simulink model "IEEE34_PQload"  (R2021b)
settings: Solver=ode4  StartTime=0.0  StopTime=5  FixedStep=50e-6  RelTol=1e-3
PreLoadFcn:
  | pGain = 0.05; % Gain of random perturbation (pu)
  | pGainAP = 0.01; % Gain of sinusoidal active power variation (pu)
  | pGainRP = 0.01; % Gain of sinusoidal reactive power variation (pu)
  | pFreqAP = 0.03; % Frequency of sinusoidal active power variation (Hz)
  | pFreqRP = 0.03; % Frequency of sinusoidal reactive power variation (Hz)
  | 
  | init_IEEE34nodetestfeeder;
InitFcn:
  | pGain = 0.05; % Gain of random perturbation (pu)
  | pGainAP = 0.01; % Gain of sinusoidal active power variation (pu)
  | pGainRP = 0.01; % Gain of sinusoidal reactive power variation (pu)
  | pFreqAP = 0.03; % Frequency of sinusoidal active power variation (Hz)
  | pFreqRP = 0.03; % Frequency of sinusoidal reactive power variation (Hz)
  | 
  | init_IEEE34nodetestfeeder;
values from neighbouring files (symbols this model uses):
  fNom = f    (= 60)    [init_IEEE34nodetestfeeder.m]
  loadcoeff = 1.0    (= 1)    [init_IEEE34nodetestfeeder.m]
  Pbase = 500e3    (= 500000)    [init_IEEE34nodetestfeeder.m]
  Ts = 50e-6    (= 5e-05)    [init_IEEE34nodetestfeeder.m]
  vNomMV = VsubL    (= 24900)    [init_IEEE34nodetestfeeder.m]
  VsubL = 24.9e3    (= 24900)    [init_IEEE34nodetestfeeder.m]
undefined symbols (not defined in the file or in its folder): find_system
libraries: spsSeriesRLCBranchLib x330, spsGroundLib x242, LoadLib x88, spsThreePhaseVIMeasurementLib x37, spsMutualInductanceLib x24, spsVoltageMeasurementLib x18, spsCurrentMeasurementLib x12, spsOnDelayLib x12, spsRMSLib x8, spsLinearTransformerLib x6, spsControlledCurrentSourceLib x6, spsControlledVoltageSourceLib x6
(part 1 of 8)
settings Model: ARTEMISmethode_block_infos=$$__separator__$$  Creator=hosseinh  LastModifiedBy=gl8300
settings SolverCC: AlgebraicLoopSolver=TrustRegion  AutoInsertRateTranBlk=on  InsertRTBMode=Never (minimum delay)
settings DataIOCC: LimitDataPoints=on  SaveFormat=Array  SignalLoggingSaveFormat=ModelDataLogs  SaveOutput=off  SignalLogging=off  DSMLogging=off  SaveTime=off  ReturnWorkspaceOutputs=off
settings OptimizationCC: BlockReduction=off  ExpressionDepthLimit=2147483647  LifeSpan=inf
settings DebuggingCC: UnderspecifiedInitializationDetection=Classic  MergeDetectMultiDrivingBlocksExec=none  SolverPrmCheckMsg=warning  FcnCallInpInsideContextMsg=warning  AllowSymbolicDim=off  StateNameClashWarn=warning  SFUnexpectedBacktrackingDiag=warning  SFNoUnconditionalDefaultTransitionDiag=warning  SFExecutionAtInitializationDiag=none  SFMachineParentedDataDiag=warning  ArithmeticOperatorsInVariantConditions=warning
settings HardwareCC: ProdBitPerPointer=32  ProdBitPerSizeT=32  ProdBitPerPtrDiffT=32  ProdLargestAtomicFloat=None  ProdIntDivRoundTo=Undefined  ProdEndianess=Unspecified  ProdWordSize=32  ProdHWDeviceType=32-bit Generic
settings ModelReferenceCC: PropagateSignalLabelsOutOfModel=off
settings SFSimCC: SimUseLocalCustomCode=off  CustomCodeUndefinedFunction=UseInterfaceOnly
settings RTWCC: RTWUseLocalCustomCode=off
settings CodeAppCC: StateflowObjectComments=on
settings GRTTargetCC: TargetLangStandard=C89/C90 (ANSI)  CombineOutputUpdateFcns=off  GRTInterface=on
settings ConfigComp: CovMetricSettings=dw  CovSaveCumulativeToWorkspaceVar=on  CovSaveSingleToWorkspaceVar=on  CovExternalEMLEnable=off
settings SimscapeCC: SimscapeNormalizeSystem=off

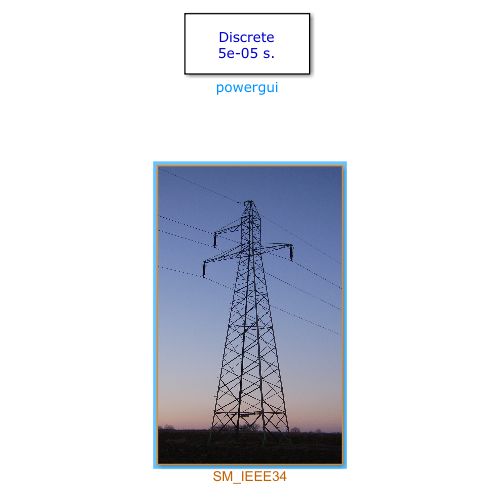
[thumbnail: Simulink's stored preview of the top-level diagram]
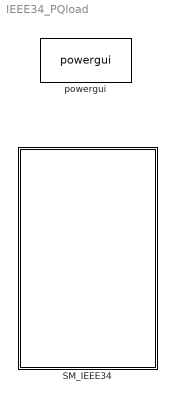
== system IEEE34_PQload ==
  SM_IEEE34 : Subsystem
      mask Display: image(imread('MVT.jpg'))
  powergui : spspowerguiLib/powergui  Priority=1  SimulationMode=Discrete  SampleTime=Ts  frequency=60  Iterations=50  frequencyindice=0  Pbase=100e6  ErrMax=1e-4  UnitsV=kV  UnitsW=MW  buscounter=0  FunctionMessages=off  echomessages=on  EnableUseOfTLC=off  CurrentSourceSwitches=off  DisableSnubberDevices=off  DisableRonSwitches=off  DisableVfSwitches=off  DisplayEquations=off  AutomaticDiscreteSolvers=off  SolverType=Backward Euler  Interpol=off  ExternalGateDelay=off  methode=off  Ts=0  x0status=blocks  SPID=off  SwTol=0  HookPort=off  NonlinearTolerance=1e-4  nMaxIteration=100  ContinueOnMaxIteration=off  RestoreLinks=warning  ResistiveCurrentMeasurement=off  Frange=[0:2:500]  Ylog=off  Xlog=on  ShowGrid=off  save=off  variable=ZData  structure=0  ZoomFFT=off  StartTime=0.0  cycles=1  DisplayStyle=1  fundamental=60  FreqAxis=off  MaxFrequency=1000  frequencyindicesteady=1  RmsSteady=1  display=off

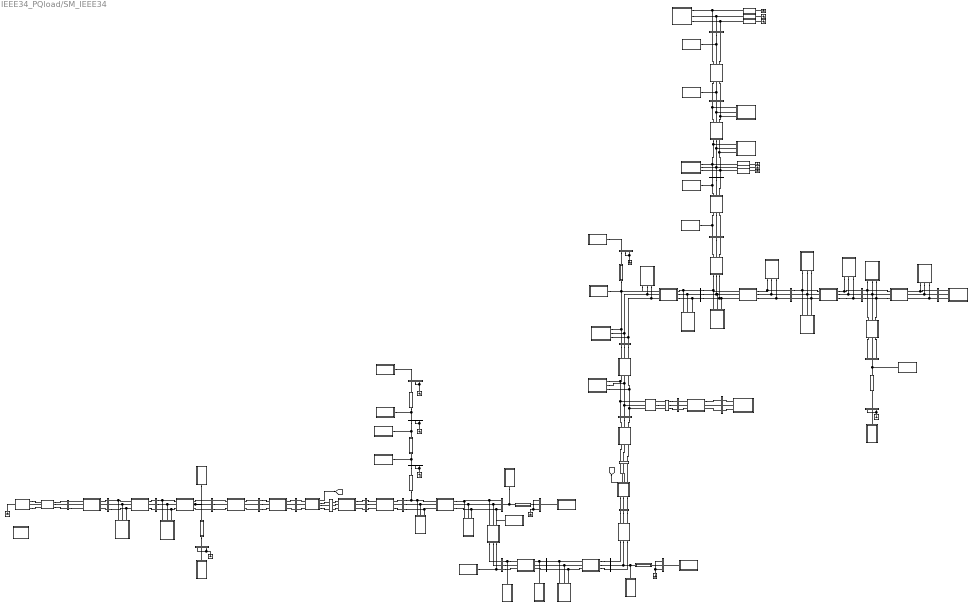
== system IEEE34_PQload/SM_IEEE34 ==
  note: Y-Z
  note: Y-PQ
  note: Y-I
  note: Y-PQ
  note: D-I
  note: Y-PQ
  note: Y-PQ
  note: Y-PQ
  note: Y-PQ
  note: D-PQ
  note: D-I
  note: Y-PQ
  note: Y-PQ
  note: Y-PQ
  note: D-I
  note: D-Z
  note: D-I
  note: Y-PQ
  note: D-PQ
  note: Y-I
  note: Y-I
  note: Y-PQ
  note: Y-Z
  800 : spsThreePhaseVIMeasurementLib/Three-Phase V-I Measurement  VoltageMeasurement=phase-to-ground  SetLabelV=on  LabelV=Vabc_800  Vpu=off  VpuLL=off  CurrentMeasurement=yes  SetLabelI=on  LabelI=Iabc_800  Ipu=off  Pbase=Pbase  Vbase=Vbase  OutputType=Complex  PhasorSimulation=off  PSBequivalent=0
  802 : spsThreePhaseVIMeasurementLib/Three-Phase V-I Measurement  VoltageMeasurement=phase-to-ground  SetLabelV=on  LabelV=Vabc_802  Vpu=off  VpuLL=off  CurrentMeasurement=yes  SetLabelI=on  LabelI=Iabc_802  Ipu=off  Pbase=Pbase  Vbase=Vbase  OutputType=Complex  PhasorSimulation=off  PSBequivalent=0
  806 : spsThreePhaseVIMeasurementLib/Three-Phase V-I Measurement  VoltageMeasurement=phase-to-ground  SetLabelV=on  LabelV=Vabc_806  Vpu=off  VpuLL=off  CurrentMeasurement=yes  SetLabelI=on  LabelI=Iabc_806  Ipu=off  Pbase=Pbase  Vbase=Vbase  OutputType=Complex  PhasorSimulation=off  PSBequivalent=0
  808 : spsThreePhaseVIMeasurementLib/Three-Phase V-I Measurement  VoltageMeasurement=phase-to-ground  SetLabelV=on  LabelV=Vabc_808  Vpu=off  VpuLL=off  CurrentMeasurement=yes  SetLabelI=on  LabelI=Iabc_808  Ipu=off  Pbase=Pbase  Vbase=Vbase  OutputType=Complex  PhasorSimulation=off  PSBequivalent=0
  810 : spsThreePhaseVIMeasurementLib/Three-Phase V-I Measurement  VoltageMeasurement=phase-to-ground  SetLabelV=on  LabelV=Vabc_810  Vpu=off  VpuLL=off  CurrentMeasurement=yes  SetLabelI=on  LabelI=Iabc_810  Ipu=off  Pbase=Pbase  Vbase=Vbase  OutputType=Complex  PhasorSimulation=off  PSBequivalent=0
  812 : spsThreePhaseVIMeasurementLib/Three-Phase V-I Measurement  VoltageMeasurement=phase-to-ground  SetLabelV=on  LabelV=Vabc_812  Vpu=off  VpuLL=off  CurrentMeasurement=yes  SetLabelI=on  LabelI=Iabc_812  Ipu=off  Pbase=Pbase  Vbase=Vbase  OutputType=Complex  PhasorSimulation=off  PSBequivalent=0
  814 : spsThreePhaseVIMeasurementLib/Three-Phase V-I Measurement  VoltageMeasurement=phase-to-ground  SetLabelV=on  LabelV=Vabc_814  Vpu=off  VpuLL=off  CurrentMeasurement=yes  SetLabelI=on  LabelI=Iabc_814  Ipu=off  Pbase=Pbase  Vbase=Vbase  OutputType=Complex  PhasorSimulation=off  PSBequivalent=0
  816 : spsThreePhaseVIMeasurementLib/Three-Phase V-I Measurement  VoltageMeasurement=phase-to-ground  SetLabelV=on  LabelV=Vabc_816  Vpu=off  VpuLL=off  CurrentMeasurement=yes  SetLabelI=on  LabelI=Iabc_816  Ipu=off  Pbase=Pbase  Vbase=Vbase  OutputType=Complex  PhasorSimulation=off  PSBequivalent=0
  818 : spsThreePhaseVIMeasurementLib/Three-Phase V-I Measurement  VoltageMeasurement=phase-to-ground  SetLabelV=on  LabelV=Vabc_818  Vpu=off  VpuLL=off  CurrentMeasurement=yes  SetLabelI=on  LabelI=Iabc_818  Ipu=off  Pbase=Pbase  Vbase=Vbase  OutputType=Complex  PhasorSimulation=off  PSBequivalent=0
  820 : spsThreePhaseVIMeasurementLib/Three-Phase V-I Measurement  VoltageMeasurement=phase-to-ground  SetLabelV=on  LabelV=Vabc_820  Vpu=off  VpuLL=off  CurrentMeasurement=yes  SetLabelI=on  LabelI=Iabc_820  Ipu=off  Pbase=Pbase  Vbase=Vbase  OutputType=Complex  PhasorSimulation=off  PSBequivalent=0
  822 : spsThreePhaseVIMeasurementLib/Three-Phase V-I Measurement  VoltageMeasurement=phase-to-ground  SetLabelV=on  LabelV=Vabc_822  Vpu=off  VpuLL=off  CurrentMeasurement=yes  SetLabelI=on  LabelI=Iabc_822  Ipu=off  Pbase=Pbase  Vbase=Vbase  OutputType=Complex  PhasorSimulation=off  PSBequivalent=0
  824 : spsThreePhaseVIMeasurementLib/Three-Phase V-I Measurement  VoltageMeasurement=phase-to-ground  SetLabelV=on  LabelV=Vabc_824  Vpu=off  VpuLL=off  CurrentMeasurement=yes  SetLabelI=on  LabelI=Iabc_824  Ipu=off  Pbase=Pbase  Vbase=Vbase  OutputType=Complex  PhasorSimulation=off  PSBequivalent=0
  826 : spsThreePhaseVIMeasurementLib/Three-Phase V-I Measurement  VoltageMeasurement=phase-to-ground  SetLabelV=on  LabelV=Vabc_826  Vpu=off  VpuLL=off  CurrentMeasurement=yes  SetLabelI=on  LabelI=Iabc_826  Ipu=off  Pbase=Pbase  Vbase=Vbase  OutputType=Complex  PhasorSimulation=off  PSBequivalent=0
  828 : spsThreePhaseVIMeasurementLib/Three-Phase V-I Measurement  VoltageMeasurement=phase-to-ground  SetLabelV=on  LabelV=Vabc_828  Vpu=off  VpuLL=off  CurrentMeasurement=yes  SetLabelI=on  LabelI=Iabc_828  Ipu=off  Pbase=Pbase  Vbase=Vbase  OutputType=Complex  PhasorSimulation=off  PSBequivalent=0
  830 : spsThreePhaseVIMeasurementLib/Three-Phase V-I Measurement  VoltageMeasurement=phase-to-ground  SetLabelV=on  LabelV=Vabc_830  Vpu=off  VpuLL=off  CurrentMeasurement=yes  SetLabelI=on  LabelI=Iabc_830  Ipu=off  Pbase=Pbase  Vbase=Vbase  OutputType=Complex  PhasorSimulation=off  PSBequivalent=0
  832 : spsThreePhaseVIMeasurementLib/Three-Phase V-I Measurement  VoltageMeasurement=phase-to-ground  SetLabelV=on  LabelV=Vabc_832  Vpu=off  VpuLL=off  CurrentMeasurement=yes  SetLabelI=on  LabelI=Iabc_832  Ipu=off  Pbase=Pbase  Vbase=Vbase  OutputType=Complex  PhasorSimulation=off  PSBequivalent=0
  834 : spsThreePhaseVIMeasurementLib/Three-Phase V-I Measurement  VoltageMeasurement=phase-to-ground  SetLabelV=on  LabelV=Vabc_834  Vpu=off  VpuLL=off  CurrentMeasurement=yes  SetLabelI=on  LabelI=Iabc_834  Ipu=off  Pbase=Pbase  Vbase=Vbase  OutputType=Complex  PhasorSimulation=off  PSBequivalent=0
  836 : spsThreePhaseVIMeasurementLib/Three-Phase V-I Measurement  VoltageMeasurement=phase-to-ground  SetLabelV=on  LabelV=Vabc_836  Vpu=off  VpuLL=off  CurrentMeasurement=yes  SetLabelI=on  LabelI=Iabc_836  Ipu=off  Pbase=Pbase  Vbase=Vbase  OutputType=Complex  PhasorSimulation=off  PSBequivalent=0
  838 : spsThreePhaseVIMeasurementLib/Three-Phase V-I Measurement  VoltageMeasurement=phase-to-ground  SetLabelV=on  LabelV=Vabc_838  Vpu=off  VpuLL=off  CurrentMeasurement=yes  SetLabelI=on  LabelI=Iabc_838  Ipu=off  Pbase=Pbase  Vbase=Vbase  OutputType=Complex  PhasorSimulation=off  PSBequivalent=0
  840 : spsThreePhaseVIMeasurementLib/Three-Phase V-I Measurement  VoltageMeasurement=phase-to-ground  SetLabelV=on  LabelV=Vabc_840  Vpu=off  VpuLL=off  CurrentMeasurement=yes  SetLabelI=on  LabelI=Iabc_840  Ipu=off  Pbase=Pbase  Vbase=Vbase  OutputType=Complex  PhasorSimulation=off  PSBequivalent=0
  842 : spsThreePhaseVIMeasurementLib/Three-Phase V-I Measurement  VoltageMeasurement=phase-to-ground  SetLabelV=on  LabelV=Vabc_842  Vpu=off  VpuLL=off  CurrentMeasurement=yes  SetLabelI=on  LabelI=Iabc_842  Ipu=off  Pbase=Pbase  Vbase=Vbase  OutputType=Complex  PhasorSimulation=off  PSBequivalent=0
  844 : spsThreePhaseVIMeasurementLib/Three-Phase V-I Measurement  VoltageMeasurement=phase-to-ground  SetLabelV=on  LabelV=Vabc_844  Vpu=off  VpuLL=off  CurrentMeasurement=yes  SetLabelI=on  LabelI=Iabc_844  Ipu=off  Pbase=Pbase  Vbase=Vbase  OutputType=Complex  PhasorSimulation=off  PSBequivalent=0
  846 : spsThreePhaseVIMeasurementLib/Three-Phase V-I Measurement  VoltageMeasurement=phase-to-ground  SetLabelV=on  LabelV=Vabc_846  Vpu=off  VpuLL=off  CurrentMeasurement=yes  SetLabelI=on  LabelI=Iabc_846  Ipu=off  Pbase=Pbase  Vbase=Vbase  OutputType=Complex  PhasorSimulation=off  PSBequivalent=0
  848 : spsThreePhaseVIMeasurementLib/Three-Phase V-I Measurement  VoltageMeasurement=phase-to-ground  SetLabelV=on  LabelV=Vabc_848  Vpu=off  VpuLL=off  CurrentMeasurement=yes  SetLabelI=on  LabelI=Iabc_848  Ipu=off  Pbase=Pbase  Vbase=Vbase  OutputType=Complex  PhasorSimulation=off  PSBequivalent=0
  850 : spsThreePhaseVIMeasurementLib/Three-Phase V-I Measurement  VoltageMeasurement=phase-to-ground  SetLabelV=on  LabelV=Vabc_850  Vpu=off  VpuLL=off  CurrentMeasurement=yes  SetLabelI=on  LabelI=Iabc_850  Ipu=off  Pbase=Pbase  Vbase=Vbase  OutputType=Complex  PhasorSimulation=off  PSBequivalent=0
  "852 " : spsThreePhaseVIMeasurementLib/Three-Phase V-I Measurement  VoltageMeasurement=phase-to-ground  SetLabelV=on  LabelV=Vabc_852  Vpu=off  VpuLL=off  CurrentMeasurement=yes  SetLabelI=on  LabelI=Iabc_852  Ipu=off  Pbase=100e6  Vbase=24900  OutputType=Complex  PhasorSimulation=off  PSBequivalent=0
  854 : spsThreePhaseVIMeasurementLib/Three-Phase V-I Measurement  VoltageMeasurement=phase-to-ground  SetLabelV=on  LabelV=Vabc_854  Vpu=off  VpuLL=off  CurrentMeasurement=yes  SetLabelI=on  LabelI=Iabc_854  Ipu=off  Pbase=Pbase  Vbase=Vbase  OutputType=Complex  PhasorSimulation=off  PSBequivalent=0
  856 : spsThreePhaseVIMeasurementLib/Three-Phase V-I Measurement  VoltageMeasurement=phase-to-ground  SetLabelV=on  LabelV=Vabc_856  Vpu=off  VpuLL=off  CurrentMeasurement=yes  SetLabelI=on  LabelI=Iabc_856  Ipu=off  Pbase=Pbase  Vbase=Vbase  OutputType=Complex  PhasorSimulation=off  PSBequivalent=0
  858 : spsThreePhaseVIMeasurementLib/Three-Phase V-I Measurement  VoltageMeasurement=phase-to-ground  SetLabelV=on  LabelV=Vabc_858  Vpu=off  VpuLL=off  CurrentMeasurement=yes  SetLabelI=on  LabelI=Iabc_858  Ipu=off  Pbase=Pbase  Vbase=Vbase  OutputType=Complex  PhasorSimulation=off  PSBequivalent=0
  860 : spsThreePhaseVIMeasurementLib/Three-Phase V-I Measurement  VoltageMeasurement=phase-to-ground  SetLabelV=on  LabelV=Vabc_860  Vpu=off  VpuLL=off  CurrentMeasurement=yes  SetLabelI=on  LabelI=Iabc_860  Ipu=off  Pbase=Pbase  Vbase=Vbase  OutputType=Complex  PhasorSimulation=off  PSBequivalent=0
  862 : spsThreePhaseVIMeasurementLib/Three-Phase V-I Measurement  VoltageMeasurement=phase-to-ground  SetLabelV=on  LabelV=Vabc_862  Vpu=off  VpuLL=off  CurrentMeasurement=yes  SetLabelI=on  LabelI=Iabc_862  Ipu=off  Pbase=Pbase  Vbase=Vbase  OutputType=Complex  PhasorSimulation=off  PSBequivalent=0
  864 : spsThreePhaseVIMeasurementLib/Three-Phase V-I Measurement  VoltageMeasurement=phase-to-ground  SetLabelV=on  LabelV=Vabc_864  Vpu=off  VpuLL=off  CurrentMeasurement=yes  SetLabelI=on  LabelI=Iabc_864  Ipu=off  Pbase=Pbase  Vbase=Vbase  OutputType=Complex  PhasorSimulation=off  PSBequivalent=0
  888 : spsThreePhaseVIMeasurementLib/Three-Phase V-I Measurement  VoltageMeasurement=phase-to-ground  SetLabelV=on  LabelV=Vabc_888  Vpu=off  VpuLL=off  CurrentMeasurement=yes  SetLabelI=on  LabelI=Iabc_888  Ipu=off  Pbase=Pbase  Vbase=VxfmL  OutputType=Complex  PhasorSimulation=off  PSBequivalent=0
  890 : spsThreePhaseVIMeasurementLib/Three-Phase V-I Measurement  VoltageMeasurement=phase-to-ground  SetLabelV=on  LabelV=Vabc_890  Vpu=off  VpuLL=off  CurrentMeasurement=yes  SetLabelI=on  LabelI=Iabc_890  Ipu=off  Pbase=Pbase  Vbase=VxfmL  OutputType=Complex  PhasorSimulation=off  PSBequivalent=0
  Config1 : Subsystem  mask(Config302 (IEEE 34 Node Test Feeder)){fNom=fNom, length=1.6 * 48150 / 5280}
      mask prompts: fNom "Nominal frequency (Hz)"; length "Length (km)"
      mask Display:
      | patch([20 20 80 80], [30 70 70 30])
      | patch([0 0 20 20], [47 53 53 47])
      | patch([80 80 100 100], [47 53 53 47])
  Config10 : Subsystem  mask(Config300 (IEEE 34 Node Test Feeder)){fNom=fNom, length=1.6 * 29730 / 5280}
      mask prompts: fNom "Nominal frequency (Hz)"; length "Length (km)"
      mask Display:
      | patch([20 20 80 80], [0 20 20 0])
      | patch([0 0 20 20], [7 13 13 7])
      | patch([80 80 100 100], [7 13 13 7])
      | 
      | patch([20 20 80 80], [40 60 60 40])
      | patch([0 0 20 20], [47 53 53 47])
      | patch([80 80 100 100], [47 53 53 47])
      | 
      | patch([20 20 80 80], [80 100 100 80])
      | patch([0 0 20 20], [87 93 93 87])
      | patch([80 80 100 100], [87 93 93 87])
  Config11 : Subsystem  mask(Config301 (IEEE 34 Node Test Feeder)){fNom=fNom, length=1.6 * 310 / 5280}
      mask prompts: fNom "Nominal frequency (Hz)"; length "Length (km)"
      mask Display:
      | patch([20 20 80 80], [0 20 20 0])
      | patch([0 0 20 20], [7 13 13 7])
      | patch([80 80 100 100], [7 13 13 7])
      | 
      | patch([20 20 80 80], [40 60 60 40])
      | patch([0 0 20 20], [47 53 53 47])
      | patch([80 80 100 100], [47 53 53 47])
      | 
      | patch([20 20 80 80], [80 100 100 80])
      | patch([0 0 20 20], [87 93 93 87])
      | patch([80 80 100 100], [87 93 93 87])
  Config12 : Subsystem  mask(Config301 (IEEE 34 Node Test Feeder)){fNom=fNom, length=1.6 * 10210 / 5280}
      mask prompts: fNom "Nominal frequency (Hz)"; length "Length (km)"
      mask Display:
      | patch([20 20 80 80], [0 20 20 0])
      | patch([0 0 20 20], [7 13 13 7])
      | patch([80 80 100 100], [7 13 13 7])
      | 
      | patch([20 20 80 80], [40 60 60 40])
      | patch([0 0 20 20], [47 53 53 47])
      | patch([80 80 100 100], [47 53 53 47])
      | 
      | patch([20 20 80 80], [80 100 100 80])
      | patch([0 0 20 20], [87 93 93 87])
      | patch([80 80 100 100], [87 93 93 87])
  Config13 : Subsystem  mask(Config300 (IEEE 34 Node Test Feeder)){fNom=fNom, length=1.6 * 10560 / 5280}
      mask prompts: fNom "Nominal frequency (Hz)"; length "Length (km)"
      mask Display:
      | patch([20 20 80 80], [0 20 20 0])
      | patch([0 0 20 20], [7 13 13 7])
      | patch([80 80 100 100], [7 13 13 7])
      | 
      | patch([20 20 80 80], [40 60 60 40])
      | patch([0 0 20 20], [47 53 53 47])
      | patch([80 80 100 100], [47 53 53 47])
      | 
      | patch([20 20 80 80], [80 100 100 80])
      | patch([0 0 20 20], [87 93 93 87])
      | patch([80 80 100 100], [87 93 93 87])
  Config14 : Subsystem  mask(Config301 (IEEE 34 Node Test Feeder)){fNom=fNom, length=1.6 * 20440 / 5280}
      mask prompts: fNom "Nominal frequency (Hz)"; length "Length (km)"
      mask Display:
      | patch([20 20 80 80], [0 20 20 0])
      | patch([0 0 20 20], [7 13 13 7])
      | patch([80 80 100 100], [7 13 13 7])
      | 
      | patch([20 20 80 80], [40 60 60 40])
      | patch([0 0 20 20], [47 53 53 47])
      | patch([80 80 100 100], [47 53 53 47])
      | 
      | patch([20 20 80 80], [80 100 100 80])
      | patch([0 0 20 20], [87 93 93 87])
      | patch([80 80 100 100], [87 93 93 87])
  Config15 : Subsystem  mask(Config301 (IEEE 34 Node Test Feeder)){fNom=fNom, length=1.6 * 520 / 5280}
      mask prompts: fNom "Nominal frequency (Hz)"; length "Length (km)"
      mask Display:
      | patch([20 20 80 80], [0 20 20 0])
      | patch([0 0 20 20], [7 13 13 7])
      | patch([80 80 100 100], [7 13 13 7])
      | 
      | patch([20 20 80 80], [40 60 60 40])
      | patch([0 0 20 20], [47 53 53 47])
      | patch([80 80 100 100], [47 53 53 47])
      | 
      | patch([20 20 80 80], [80 100 100 80])
      | patch([0 0 20 20], [87 93 93 87])
      | patch([80 80 100 100], [87 93 93 87])
  Config16 : Subsystem  mask(Config301 (IEEE 34 Node Test Feeder)){fNom=fNom, length=1.6 * 36830 / 5280}
      mask prompts: fNom "Nominal frequency (Hz)"; length "Length (km)"
      mask Display:
      | patch([20 20 80 80], [0 20 20 0])
      | patch([0 0 20 20], [7 13 13 7])
      | patch([80 80 100 100], [7 13 13 7])
      | 
      | patch([20 20 80 80], [40 60 60 40])
      | patch([0 0 20 20], [47 53 53 47])
      | patch([80 80 100 100], [47 53 53 47])
      | 
      | patch([20 20 80 80], [80 100 100 80])
      | patch([0 0 20 20], [87 93 93 87])
      | patch([80 80 100 100], [87 93 93 87])
  Config17 : Subsystem  mask(Config301 (IEEE 34 Node Test Feeder)){fNom=fNom, length=1.6 * 4900 / 5280}
      mask prompts: fNom "Nominal frequency (Hz)"; length "Length (km)"
      mask Display:
      | patch([20 20 80 80], [0 20 20 0])
      | patch([0 0 20 20], [7 13 13 7])
      | patch([80 80 100 100], [7 13 13 7])
      | 
      | patch([20 20 80 80], [40 60 60 40])
      | patch([0 0 20 20], [47 53 53 47])
      | patch([80 80 100 100], [47 53 53 47])
      | 
      | patch([20 20 80 80], [80 100 100 80])
      | patch([0 0 20 20], [87 93 93 87])
      | patch([80 80 100 100], [87 93 93 87])
  Config18 : Subsystem  mask(Config301 (IEEE 34 Node Test Feeder)){fNom=fNom, length=1.6 * 280 / 5280}
      mask prompts: fNom "Nominal frequency (Hz)"; length "Length (km)"
      mask Display:
      | patch([20 20 80 80], [0 20 20 0])
      | patch([0 0 20 20], [7 13 13 7])
      | patch([80 80 100 100], [7 13 13 7])
      | 
      | patch([20 20 80 80], [40 60 60 40])
      | patch([0 0 20 20], [47 53 53 47])
      | patch([80 80 100 100], [47 53 53 47])
      | 
      | patch([20 20 80 80], [80 100 100 80])
      | patch([0 0 20 20], [87 93 93 87])
      | patch([80 80 100 100], [87 93 93 87])
  Config19 : Subsystem  mask(Config301 (IEEE 34 Node Test Feeder)){fNom=fNom, length=1.6 * 1350 / 5280}
      mask prompts: fNom "Nominal frequency (Hz)"; length "Length (km)"
      mask Display:
      | patch([20 20 80 80], [0 20 20 0])
      | patch([0 0 20 20], [7 13 13 7])
      | patch([80 80 100 100], [7 13 13 7])
      | 
      | patch([20 20 80 80], [40 60 60 40])
      | patch([0 0 20 20], [47 53 53 47])
      | patch([80 80 100 100], [47 53 53 47])
      | 
      | patch([20 20 80 80], [80 100 100 80])
      | patch([0 0 20 20], [87 93 93 87])
      | patch([80 80 100 100], [87 93 93 87])
  Config2 : Subsystem  mask(Config302 (IEEE 34 Node Test Feeder)){fNom=fNom, length=1.6 * 13740 / 5280}
      mask prompts: fNom "Nominal frequency (Hz)"; length "Length (km)"
      mask Display:
      | patch([20 20 80 80], [30 70 70 30])
      | patch([0 0 20 20], [47 53 53 47])
      | patch([80 80 100 100], [47 53 53 47])
  Config20 : Subsystem  mask(Config301 (IEEE 34 Node Test Feeder)){fNom=fNom, length=1.6 * 3640 / 5280}
      mask prompts: fNom "Nominal frequency (Hz)"; length "Length (km)"
      mask Display:
      | patch([20 20 80 80], [0 20 20 0])
      | patch([0 0 20 20], [7 13 13 7])
      | patch([80 80 100 100], [7 13 13 7])
      | 
      | patch([20 20 80 80], [40 60 60 40])
      | patch([0 0 20 20], [47 53 53 47])
      | patch([80 80 100 100], [47 53 53 47])
      | 
      | patch([20 20 80 80], [80 100 100 80])
      | patch([0 0 20 20], [87 93 93 87])
      | patch([80 80 100 100], [87 93 93 87])
  Config21 : Subsystem  mask(Config301 (IEEE 34 Node Test Feeder)){fNom=fNom, length=1.6 * 2020 / 5280}
      mask prompts: fNom "Nominal frequency (Hz)"; length "Length (km)"
      mask Display:
      | patch([20 20 80 80], [0 20 20 0])
      | patch([0 0 20 20], [7 13 13 7])
      | patch([80 80 100 100], [7 13 13 7])
      | 
      | patch([20 20 80 80], [40 60 60 40])
      | patch([0 0 20 20], [47 53 53 47])
      | patch([80 80 100 100], [47 53 53 47])
      | 
      | patch([20 20 80 80], [80 100 100 80])
      | patch([0 0 20 20], [87 93 93 87])
      | patch([80 80 100 100], [87 93 93 87])
  Config22 : Subsystem  mask(Config301 (IEEE 34 Node Test Feeder)){fNom=fNom, length=1.6 * 2680 / 5280}
      mask prompts: fNom "Nominal frequency (Hz)"; length "Length (km)"
      mask Display:
      | patch([20 20 80 80], [0 20 20 0])
      | patch([0 0 20 20], [7 13 13 7])
      | patch([80 80 100 100], [7 13 13 7])
      | 
      | patch([20 20 80 80], [40 60 60 40])
      | patch([0 0 20 20], [47 53 53 47])
      | patch([80 80 100 100], [47 53 53 47])
      | 
      | patch([20 20 80 80], [80 100 100 80])
      | patch([0 0 20 20], [87 93 93 87])
      | patch([80 80 100 100], [87 93 93 87])
  Config23 : Subsystem  mask(Config301 (IEEE 34 Node Test Feeder)){fNom=fNom, length=1.6 * 530 / 5280}
      mask prompts: fNom "Nominal frequency (Hz)"; length "Length (km)"
      mask Display:
      | patch([20 20 80 80], [0 20 20 0])
      | patch([0 0 20 20], [7 13 13 7])
      | patch([80 80 100 100], [7 13 13 7])
      | 
      | patch([20 20 80 80], [40 60 60 40])
      | patch([0 0 20 20], [47 53 53 47])
      | patch([80 80 100 100], [47 53 53 47])
      | 
      | patch([20 20 80 80], [80 100 100 80])
      | patch([0 0 20 20], [87 93 93 87])
      | patch([80 80 100 100], [87 93 93 87])
  Config24 : Subsystem  mask(Config301 (IEEE 34 Node Test Feeder)){fNom=fNom, length=1.6 * 5830 / 5280}
      mask prompts: fNom "Nominal frequency (Hz)"; length "Length (km)"
      mask Display:
      | patch([20 20 80 80], [0 20 20 0])
      | patch([0 0 20 20], [7 13 13 7])
      | patch([80 80 100 100], [7 13 13 7])
      | 
      | patch([20 20 80 80], [40 60 60 40])
      | patch([0 0 20 20], [47 53 53 47])
      | patch([80 80 100 100], [47 53 53 47])
      | 
      | patch([20 20 80 80], [80 100 100 80])
      | patch([0 0 20 20], [87 93 93 87])
      | patch([80 80 100 100], [87 93 93 87])
  Config25 : Subsystem  mask(Config301 (IEEE 34 Node Test Feeder)){fNom=fNom, length=1.6 * 860 / 5280}
      mask prompts: fNom "Nominal frequency (Hz)"; length "Length (km)"
      mask Display:
      | patch([20 20 80 80], [0 20 20 0])
      | patch([0 0 20 20], [7 13 13 7])
      | patch([80 80 100 100], [7 13 13 7])
      | 
      | patch([20 20 80 80], [40 60 60 40])
      | patch([0 0 20 20], [47 53 53 47])
      | patch([80 80 100 100], [47 53 53 47])
      | 
      | patch([20 20 80 80], [80 100 100 80])
      | patch([0 0 20 20], [87 93 93 87])
      | patch([80 80 100 100], [87 93 93 87])
  Config26 : Subsystem  mask(Config301 (IEEE 34 Node Test Feeder)){fNom=fNom, length=1.6 * 280 / 5280}
      mask prompts: fNom "Nominal frequency (Hz)"; length "Length (km)"
      mask Display:
      | patch([20 20 80 80], [0 20 20 0])
      | patch([0 0 20 20], [7 13 13 7])
      | patch([80 80 100 100], [7 13 13 7])
      | 
      | patch([20 20 80 80], [40 60 60 40])
      | patch([0 0 20 20], [47 53 53 47])
      | patch([80 80 100 100], [47 53 53 47])
      | 
      | patch([20 20 80 80], [80 100 100 80])
      | patch([0 0 20 20], [87 93 93 87])
      | patch([80 80 100 100], [87 93 93 87])
  Config27 : Subsystem  mask(Config301 (IEEE 34 Node Test Feeder)){fNom=fNom, length=1.6 * 840 / 5280}
      mask prompts: fNom "Nominal frequency (Hz)"; length "Length (km)"
      mask Display:
      | patch([20 20 80 80], [0 20 20 0])
      | patch([0 0 20 20], [7 13 13 7])
      | patch([80 80 100 100], [7 13 13 7])
      | 
      | patch([20 20 80 80], [40 60 60 40])
      | patch([0 0 20 20], [47 53 53 47])
      | patch([80 80 100 100], [47 53 53 47])
      | 
      | patch([20 20 80 80], [80 100 100 80])
      | patch([0 0 20 20], [87 93 93 87])
      | patch([80 80 100 100], [87 93 93 87])
  Config3 : Subsystem  mask(Config303 (IEEE 34 Node Test Feeder)){fNom=fNom, length=1.6 * 3030 / 5280}
      mask prompts: fNom "Nominal frequency (Hz)"; length "Length (km)"
      mask Display:
      | patch([20 20 80 80], [30 70 70 30])
      | patch([0 0 20 20], [47 53 53 47])
      | patch([80 80 100 100], [47 53 53 47])
  Config300 : Subsystem  mask(Config300 (IEEE 34 Node Test Feeder)){fNom=fNom, length=1.6 * 2580 / 5280}
      mask prompts: fNom "Nominal frequency (Hz)"; length "Length (km)"
      mask Display:
      | patch([20 20 80 80], [0 20 20 0])
      | patch([0 0 20 20], [7 13 13 7])
      | patch([80 80 100 100], [7 13 13 7])
      | 
      | patch([20 20 80 80], [40 60 60 40])
      | patch([0 0 20 20], [47 53 53 47])
      | patch([80 80 100 100], [47 53 53 47])
      | 
      | patch([20 20 80 80], [80 100 100 80])
      | patch([0 0 20 20], [87 93 93 87])
      | patch([80 80 100 100], [87 93 93 87])
  Config301 : Subsystem  mask(Config301 (IEEE 34 Node Test Feeder)){fNom=fNom, length=1.6 * 10 / 5280}
      mask prompts: fNom "Nominal frequency (Hz)"; length "Length (km)"
      mask Display:
      | patch([20 20 80 80], [0 20 20 0])
      | patch([0 0 20 20], [7 13 13 7])
      | patch([80 80 100 100], [7 13 13 7])
      | 
      | patch([20 20 80 80], [40 60 60 40])
      | patch([0 0 20 20], [47 53 53 47])
      | patch([80 80 100 100], [47 53 53 47])
      | 
      | patch([20 20 80 80], [80 100 100 80])
      | patch([0 0 20 20], [87 93 93 87])
      | patch([80 80 100 100], [87 93 93 87])
  Config302 : Subsystem  mask(Config302 (IEEE 34 Node Test Feeder)){fNom=fNom, length=1.6 * 1710 / 5280}
      mask prompts: fNom "Nominal frequency (Hz)"; length "Length (km)"
      mask Display:
      | patch([20 20 80 80], [30 70 70 30])
      | patch([0 0 20 20], [47 53 53 47])
      | patch([80 80 100 100], [47 53 53 47])
  Config303 : Subsystem  mask(Config303 (IEEE 34 Node Test Feeder)){fNom=fNom, length=1.6 * 5804 / 5280}
      mask prompts: fNom "Nominal frequency (Hz)"; length "Length (km)"
      mask Display:
      | patch([20 20 80 80], [30 70 70 30])
      | patch([0 0 20 20], [47 53 53 47])
      | patch([80 80 100 100], [47 53 53 47])
  Config304 : Subsystem  mask(Config304 (IEEE 34 Node Test Feeder)){fNom=fNom, length=1.6 * 4860 / 5280}
      mask prompts: fNom "Nominal frequency (Hz)"; length "Length (km)"
      mask Display:
      | patch([20 20 80 80], [30 70 70 30])
      | patch([0 0 20 20], [47 53 53 47])
      | patch([80 80 100 100], [47 53 53 47])
  Config4 : Subsystem  mask(Config303 (IEEE 34 Node Test Feeder)){fNom=fNom, length=1.6 * 3030 / 5280}
      mask prompts: fNom "Nominal frequency (Hz)"; length "Length (km)"
      mask Display:
      | patch([20 20 80 80], [30 70 70 30])
      | patch([0 0 20 20], [47 53 53 47])
      | patch([80 80 100 100], [47 53 53 47])
  Config5 : Subsystem  mask(Config301 (IEEE 34 Node Test Feeder)){fNom=fNom, length=1.6 * 10 / 5280}
      mask prompts: fNom "Nominal frequency (Hz)"; length "Length (km)"
      mask Display:
      | patch([20 20 80 80], [0 20 20 0])
      | patch([0 0 20 20], [7 13 13 7])
      | patch([80 80 100 100], [7 13 13 7])
      | 
      | patch([20 20 80 80], [40 60 60 40])
      | patch([0 0 20 20], [47 53 53 47])
      | patch([80 80 100 100], [47 53 53 47])
      | 
      | patch([20 20 80 80], [80 100 100 80])
      | patch([0 0 20 20], [87 93 93 87])
      | patch([80 80 100 100], [87 93 93 87])
  Config6 : Subsystem  mask(Config302 (IEEE 34 Node Test Feeder)){fNom=fNom, length=1.6 * 1620 / 5280}
      mask prompts: fNom "Nominal frequency (Hz)"; length "Length (km)"
      mask Display:
      | patch([20 20 80 80], [30 70 70 30])
      | patch([0 0 20 20], [47 53 53 47])
      | patch([80 80 100 100], [47 53 53 47])
  Config7 : Subsystem  mask(Config300 (IEEE 34 Node Test Feeder)){fNom=fNom, length=1.6 * 1730 / 5280}
      mask prompts: fNom "Nominal frequency (Hz)"; length "Length (km)"
      mask Display:
      | patch([20 20 80 80], [0 20 20 0])
      | patch([0 0 20 20], [7 13 13 7])
      | patch([80 80 100 100], [7 13 13 7])
      | 
      | patch([20 20 80 80], [40 60 60 40])
      | patch([0 0 20 20], [47 53 53 47])
      | patch([80 80 100 100], [47 53 53 47])
      | 
      | patch([20 20 80 80], [80 100 100 80])
      | patch([0 0 20 20], [87 93 93 87])
      | patch([80 80 100 100], [87 93 93 87])
  Config8 : Subsystem  mask(Config300 (IEEE 34 Node Test Feeder)){fNom=fNom, length=1.6 * 32230 / 5280}
      mask prompts: fNom "Nominal frequency (Hz)"; length "Length (km)"
      mask Display:
      | patch([20 20 80 80], [0 20 20 0])
      | patch([0 0 20 20], [7 13 13 7])
      | patch([80 80 100 100], [7 13 13 7])
      | 
      | patch([20 20 80 80], [40 60 60 40])
      | patch([0 0 20 20], [47 53 53 47])
      | patch([80 80 100 100], [47 53 53 47])
      | 
      | patch([20 20 80 80], [80 100 100 80])
      | patch([0 0 20 20], [87 93 93 87])
      | patch([80 80 100 100], [87 93 93 87])
  Config9 : Subsystem  mask(Config300 (IEEE 34 Node Test Feeder)){fNom=fNom, length=1.6 * 37500 / 5280}
      mask prompts: fNom "Nominal frequency (Hz)"; length "Length (km)"
      mask Display:
      | patch([20 20 80 80], [0 20 20 0])
      | patch([0 0 20 20], [7 13 13 7])
      | patch([80 80 100 100], [7 13 13 7])
      | 
      | patch([20 20 80 80], [40 60 60 40])
      | patch([0 0 20 20], [47 53 53 47])
      | patch([80 80 100 100], [47 53 53 47])
      | 
      | patch([20 20 80 80], [80 100 100 80])
      | patch([0 0 20 20], [87 93 93 87])
      | patch([80 80 100 100], [87 93 93 87])
  DL_802 : Subsystem
  DL_806 : Subsystem
  DL_808 : Subsystem
  DL_810 : Subsystem
  DL_816 D I : Subsystem
  DL_818 : Subsystem
  DL_820 : Subsystem
  DL_820 Y PQ : Subsystem
  DL_822 : Subsystem
  DL_824 D I : Subsystem
  DL_824 D-I : Subsystem
  DL_824 Y-PQ : Subsystem
  DL_826 : Subsystem
  DL_828 : Subsystem
  DL_828 Y-PQ : Subsystem
  DL_830 Y-PQ : Subsystem
  DL_832 D-Z : Subsystem
  DL_834 D-PQ : Subsystem
  DL_834 D-Z : Subsystem
  DL_836 D-I : Subsystem
  DL_836-840 : Subsystem
  DL_842 Y-PQ : Subsystem
  DL_842-844 : Subsystem
  DL_844 Y-PQ : Subsystem
  DL_846 Y-PQ : Subsystem
  DL_846 Y-PQ1 : Subsystem
  DL_848 Y-PQ : Subsystem
  DL_854 Y-PQ : Subsystem
  DL_856 : Subsystem
  DL_858 D-PQ : Subsystem
  DL_858 D-Z : Subsystem
  DL_858 Y-PQ : Subsystem
  DL_858-864 : Subsystem
  DL_860 D-PQ : Subsystem
  DL_860 D-Z : Subsystem
  DL_860-836 : Subsystem
  DL_862 Y-PQ : Subsystem
  DL_862-838 : Subsystem
  Ground{,1..12,14,22} (15 alike) : spsGroundLib/Ground  LConnTagsString=a
  Node Voltages : Subsystem
  RG10 : spsThreePhaseVIMeasurementLib/Three-Phase V-I Measurement  VoltageMeasurement=phase-to-ground  SetLabelV=on  LabelV=RG10  Vpu=off  VpuLL=off  CurrentMeasurement=yes  SetLabelI=on  LabelI=IRG10  Ipu=off  Pbase=100e6  Vbase=24900  OutputType=Complex  PhasorSimulation=off  PSBequivalent=0
  RG11 : spsThreePhaseVIMeasurementLib/Three-Phase V-I Measurement  VoltageMeasurement=phase-to-ground  SetLabelV=on  LabelV=RG11  Vpu=off  VpuLL=off  CurrentMeasurement=yes  SetLabelI=on  LabelI=IRG11  Ipu=off  Pbase=100e6  Vbase=24900  OutputType=Complex  PhasorSimulation=off  PSBequivalent=0
  Regulator 1 : Subsystem
  Regulator 2 : Subsystem
  Shunt Capacitor : spsSeriesRLCLoadLib/Series RLC Load  LConnTagsString=a  RConnTagsString=__new0  NominalVoltage=vNomMV/sqrt(3)  NominalFrequency=fNom  ActivePower=0  InductivePower=0  CapacitivePower=100e3  Setx0=off  InitialVoltage=0  SetiL0=off  InitialCurrent=0  Measurements=None  LoadType=constant Z
  Shunt Capacitor1 : spsSeriesRLCLoadLib/Series RLC Load  LConnTagsString=a  RConnTagsString=__new0  NominalVoltage=vNomMV/sqrt(3)  NominalFrequency=fNom  ActivePower=0  InductivePower=0  CapacitivePower=100e3  Setx0=off  InitialVoltage=0  SetiL0=off  InitialCurrent=0  Measurements=None  LoadType=constant Z
  Shunt Capacitor2 : spsSeriesRLCLoadLib/Series RLC Load  LConnTagsString=a  RConnTagsString=__new0  NominalVoltage=vNomMV/sqrt(3)  NominalFrequency=fNom  ActivePower=0  InductivePower=0  CapacitivePower=100e3  Setx0=off  InitialVoltage=0  SetiL0=off  InitialCurrent=0  Measurements=None  LoadType=constant Z
  Shunt Capacitor3 : spsSeriesRLCLoadLib/Series RLC Load  LConnTagsString=a  RConnTagsString=__new0  NominalVoltage=vNomMV/sqrt(3)  NominalFrequency=fNom  ActivePower=0  InductivePower=0  CapacitivePower=150e3  Setx0=off  InitialVoltage=0  SetiL0=off  InitialCurrent=0  Measurements=None  LoadType=constant Z
  Shunt Capacitor4 : spsSeriesRLCLoadLib/Series RLC Load  LConnTagsString=a  RConnTagsString=__new0  NominalVoltage=vNomMV/sqrt(3)  NominalFrequency=fNom  ActivePower=0  InductivePower=0  CapacitivePower=150e3  Setx0=off  InitialVoltage=0  SetiL0=off  InitialCurrent=0  Measurements=None  LoadType=constant Z
  Shunt Capacitor5 : spsSeriesRLCLoadLib/Series RLC Load  LConnTagsString=a  RConnTagsString=__new0  NominalVoltage=vNomMV/sqrt(3)  NominalFrequency=fNom  ActivePower=0  InductivePower=0  CapacitivePower=150e3  Setx0=off  InitialVoltage=0  SetiL0=off  InitialCurrent=0  Measurements=None  LoadType=constant Z
  Spot 830 : Subsystem
  Spot 840 : Subsystem
  Spot 844 : Subsystem
  Spot 848 : Subsystem
  Spot 860 : Subsystem
  Spot 890 : Subsystem
  Three-Phase Programmable Voltage Source : spsThreePhaseProgrammableVoltageSourceLib/Three-Phase Programmable Voltage Source  PositiveSequence="[24.9e3*1.05  0 60]"  VariationEntity=None  VariationType=Table of time-amplitude pairs  VariationTypeAlt=Step  VariationStep=0.5  VariationRate=10  VariationMagnitude=0.3  VariationFrequency=2  VariationTiming=[1 2]  VariationPhaseA=off  Amplitudes=[1 0.8 1.2 1.0]  TimeValues=[0 0.7 1.1 1.5]  HarmonicGeneration=off  HarmonicA=[3 0.2 -25 0]  HarmonicB=[2 0.15 35 2]  Timing="[0.05  3]"  BusType=swing  Pref=0  Qref=0  Qmin=-inf  Qmax=inf
  Three-Phase Series RLC Branch : spsThreePhaseSeriesRLCBranchLib/Three-Phase Series RLC Branch  LConnTagsString=A|B|C  RConnTagsString=A|B|C  BranchType=R  Resistance=0.001  Inductance=16.58e-3  Capacitance=1e-6  Measurements=None
  Three-Phase Transformer (Two Windings)1 : spsThreePhaseTransformerTwoWindingsLib/Three-Phase Transformer (Two Windings)  Winding1Connection=Yg  Winding2Connection=Yg  CoreType=Three single-phase transformers  SetSaturation=off  Hysteresis=off  DataFile='hysteresis'  SetInitialFlux=on  Measurements=None  UNITS=pu  NominalPower=[ 500e3 , 60 ]  Winding1=[24900 0.019 0.0408]  Winding2=[4160 1e-4 1e-3]  Rm=500  Lm=500  L0=0.5  Saturation="[0 0; 0.0 1.2; 1.0  1.52]"  InitialFluxes="[0.8  -0.4  0.4]"  BreakLoop=off  DiscreteSolver=Trapezoidal iterative  DataType=off  TransfoNumber=1
  XF10 : spsThreePhaseVIMeasurementLib/Three-Phase V-I Measurement  VoltageMeasurement=phase-to-ground  SetLabelV=on  LabelV=XF10  Vpu=off  VpuLL=off  CurrentMeasurement=yes  SetLabelI=on  LabelI=IXF10  Ipu=off  Pbase=100e6  Vbase=24900  OutputType=Complex  PhasorSimulation=off  PSBequivalent=0
  tag scope: Reg1=global, Reg2=global
  wires:
  Regulator 1/1(Tap) -> [Reg1]
  Regulator 2/1(Tap) -> [Reg2]
  connections:
  816/LConn1 -- Config11/RConn1
  806/RConn1 -- DL_806/RConn1 -- Config8/LConn1
  806/RConn2 -- DL_806/RConn2 -- Config8/LConn2
  Config8/LConn3 -- 806/RConn3 -- DL_806/RConn3
  Config8/RConn2 -- 808/LConn2 -- DL_808/RConn1 -- Config303/LConn1
  820/LConn1 -- DL_820/RConn1 -- Config1/LConn1
  Config2/LConn1 -- 822/LConn1
  Config303/RConn1 -- 810/LConn2
  816/LConn2 -- Config11/RConn2
  Config300/LConn1 -- 800/RConn1
  Config300/LConn2 -- 800/RConn2
  800/RConn3 -- Config300/LConn3
  Config7/LConn1 -- 802/RConn1 -- DL_802/RConn1
  Config7/LConn2 -- DL_802/RConn2 -- 802/RConn2
  802/RConn3 -- DL_802/RConn3 -- Config7/LConn3
  802/LConn3 -- Config300/RConn3
  802/LConn2 -- Config300/RConn2
  802/LConn1 -- Config300/RConn1
  Config7/RConn1 -- 806/LConn1
  806/LConn2 -- Config7/RConn2
  Config7/RConn3 -- 806/LConn3
  808/RConn3 -- Config9/LConn3
  808/RConn2 -- Config9/LConn2
  Config9/LConn1 -- 808/RConn1
  808/LConn1 -- Config8/RConn1
  808/LConn3 -- Config8/RConn3
  812/RConn1 -- Config10/LConn1
  812/LConn1 -- Config9/RConn1
  812/LConn2 -- Config9/RConn2
  812/RConn2 -- Config10/LConn2
  812/RConn3 -- Config10/LConn3
  812/LConn3 -- Config9/RConn3
  814/LConn2 -- Config10/RConn2
  814/LConn1 -- Config10/RConn1
  814/LConn3 -- Config10/RConn3
  850/LConn3 -- Config301/RConn3
  850/LConn2 -- Config301/RConn2
  Config301/RConn1 -- 850/LConn1
  850/RConn3 -- Config11/LConn3
  850/RConn2 -- Config11/LConn2
  850/RConn1 -- Config11/LConn1
  Config11/RConn3 -- 816/LConn3
  818/LConn1 -- Config302/LConn1
  818/RConn1 -- DL_818/RConn1 -- Config1/RConn1
  Config2/RConn1 -- DL_820 Y PQ/RConn1 -- 820/RConn1
  816/RConn2 -- DL_816 D I/RConn2 -- Config12/LConn2
  816/RConn3 -- Config12/LConn3 -- DL_816 D I/RConn3
  816/RConn1 -- Config302/RConn1 -- DL_816 D I/RConn1 -- Config12/LConn1
  Config15/RConn3 -- 854/LConn3
  Config15/RConn2 -- 854/LConn2
  Config15/RConn1 -- 854/LConn1
  Config15/LConn1 -- Spot 830/RConn1 -- 830/RConn1
  Config15/LConn2 -- Spot 830/RConn2 -- 830/RConn2
  Config15/LConn3 -- Spot 830/RConn3 -- 830/RConn3
  DL_824 D-I/RConn1 -- 824/RConn2 -- Config4/RConn1
  828/RConn2 -- Config14/LConn2
  828/RConn3 -- Config14/LConn3
  828/RConn1 -- Config14/LConn1 -- DL_828 Y-PQ/RConn1
  Config12/RConn3 -- DL_824 D I/RConn3 -- DL_824 Y-PQ/RConn1 -- Config27/LConn3 -- 824/LConn3
  824/LConn2 -- Config27/LConn2 -- DL_824 D I/RConn2 -- Config12/RConn2
  856/LConn2 -- Config3/LConn1
  Config3/RConn1 -- DL_854 Y-PQ/RConn1 -- 854/RConn2 -- Config16/RConn2
  Config4/LConn1 -- 826/LConn2
  830/LConn1 -- DL_830 Y-PQ/RConn1 -- Config14/RConn1
  830/LConn2 -- Config14/RConn2
  830/LConn3 -- Config14/RConn3
  Config27/RConn3 -- DL_828/RConn1 -- 828/LConn3
  Config12/RConn1 -- DL_824 D I/RConn1 -- Config27/LConn1 -- 824/LConn1
  Config24/RConn2 -- 834/LConn2 -- DL_834 D-PQ/RConn2
  Config24/RConn3 -- 834/LConn3 -- DL_834 D-PQ/RConn3
  Config24/RConn1 -- 834/LConn1 -- DL_834 D-PQ/RConn1
  858/LConn1 -- Config17/LConn1
  858/LConn2 -- Config17/LConn2
  858/LConn3 -- Config17/LConn3
  Config5/LConn1 -- 832/LConn1
  832/LConn2 -- Config5/LConn2
  832/LConn3 -- Config5/LConn3
  Config19/LConn1 -- DL_842-844/RConn1 -- 844/LConn1
  Config19/LConn3 -- 844/LConn3
  844/LConn2 -- Config19/LConn2
  Config20/LConn3 -- DL_846 Y-PQ/RConn3 -- 846/LConn3
  Config20/LConn2 -- DL_846 Y-PQ/RConn2 -- 846/LConn2
  Config20/RConn1 -- DL_844 Y-PQ/RConn1 -- 844/RConn1 -- Shunt Capacitor/LConn1 -- Spot 844/RConn1
  Config23/LConn1 -- 848/LConn1
  848/LConn2 -- DL_848 Y-PQ/RConn1 -- Config23/LConn2
  Config23/LConn3 -- 848/LConn3
  Config26/LConn3 -- DL_836 D-I/RConn3 -- 836/RConn3 -- Config25/LConn3
  Config26/LConn1 -- DL_836 D-I/RConn1 -- 836/RConn1 -- Config25/LConn1
  Config26/LConn2 -- DL_836 D-I/RConn2 -- 836/RConn2 -- Config25/LConn2
  Config22/LConn2 -- DL_860 D-PQ/RConn2 -- 860/RConn2 -- Spot 860/RConn2
  860/RConn1 -- DL_860 D-PQ/RConn1 -- Spot 860/RConn1 -- Config22/LConn1
  Config22/LConn3 -- DL_860 D-PQ/RConn3 -- 860/RConn3 -- Spot 860/RConn3
  864/LConn1 -- Config6/LConn1
  Config6/RConn1 -- DL_858 D-PQ/RConn1 -- Config24/LConn1 -- DL_858 Y-PQ/RConn1 -- DL_858 D-Z/RConn1 -- 858/RConn1
  832/RConn2 -- Three-Phase Transformer (Two Windings)1/LConn2 -- DL_832 D-Z/RConn2 -- Config17/RConn2
  832/RConn3 -- Three-Phase Transformer (Two Windings)1/LConn3 -- DL_832 D-Z/RConn3 -- Config17/RConn3
  832/RConn1 -- Three-Phase Transformer (Two Windings)1/LConn1 -- Config17/RConn1 -- DL_832 D-Z/RConn1
  Config20/LConn1 -- DL_846 Y-PQ/RConn1 -- 846/LConn1
  Config18/LConn3 -- 842/LConn3
  842/LConn2 -- Config18/LConn2
  Config18/LConn1 -- 842/LConn1
  842/RConn3 -- Config19/RConn3
  Config19/RConn2 -- 842/RConn2
  Config19/RConn1 -- DL_842 Y-PQ/RConn1 -- 842/RConn1
  844/RConn3 -- Shunt Capacitor2/LConn1 -- Spot 844/RConn3 -- DL_844 Y-PQ/RConn3 -- Config20/RConn3
  Config20/RConn2 -- DL_844 Y-PQ/RConn2 -- Shunt Capacitor1/LConn1 -- Spot 844/RConn2 -- 844/RConn2
  846/RConn3 -- Config23/RConn3
  846/RConn2 -- DL_846 Y-PQ1/RConn1 -- Config23/RConn2
  Config23/RConn1 -- 846/RConn1
  Config21/RConn1 -- DL_860 D-Z/RConn1 -- 860/LConn1
  Config21/RConn2 -- 860/LConn2 -- DL_860 D-Z/RConn2
  Config21/RConn3 -- 860/LConn3 -- DL_860 D-Z/RConn3
  Config22/RConn1 -- DL_860-836/RConn1 -- 836/LConn1
  Config22/RConn3 -- DL_860-836/RConn3 -- 836/LConn3
  Config22/RConn2 -- DL_860-836/RConn2 -- 836/LConn2
  Config26/RConn3 -- 862/LConn3
  862/LConn1 -- Config26/RConn1
  862/LConn2 -- Config26/RConn2
  Config304/LConn1 -- DL_862 Y-PQ/RConn1 -- 862/RConn2
  Ground/LConn1 -- Shunt Capacitor/RConn1
  Ground3/LConn1 -- Shunt Capacitor1/RConn1
  Ground4/LConn1 -- Shunt Capacitor2/RConn1
  Ground8/LConn1 -- Shunt Capacitor5/RConn1
  Ground7/LConn1 -- Shunt Capacitor4/RConn1
  Ground5/LConn1 -- Shunt Capacitor3/RConn1
  838/LConn2 -- Config304/RConn1
  840/LConn3 -- DL_836-840/RConn3 -- Config25/RConn3
  840/LConn2 -- DL_836-840/RConn2 -- Config25/RConn2
  840/LConn1 -- DL_836-840/RConn1 -- Config25/RConn1
  Three-Phase Series RLC Branch/LConn2 -- Three-Phase Programmable Voltage Source/RConn2
  Ground22/LConn1 -- Three-Phase Programmable Voltage Source/LConn1
  Three-Phase Programmable Voltage Source/RConn1 -- Three-Phase Series RLC Branch/LConn1
  Three-Phase Programmable Voltage Source/RConn3 -- Three-Phase Series RLC Branch/LConn3
  Three-Phase Series RLC Branch/RConn1 -- 800/LConn1
  Three-Phase Series RLC Branch/RConn2 -- 800/LConn2
  Three-Phase Series RLC Branch/RConn3 -- 800/LConn3
  Config27/RConn1 -- 828/LConn1
  Config27/RConn2 -- 828/LConn2
  Config24/LConn2 -- DL_858 D-PQ/RConn2 -- DL_858 D-Z/RConn2 -- 858/RConn2
  Config24/LConn3 -- DL_858 D-PQ/RConn3 -- DL_858 D-Z/RConn3 -- 858/RConn3
  Config16/RConn1 -- 854/RConn1
  Config16/RConn3 -- 854/RConn3
  890/LConn2 -- Config13/RConn2
  Config13/RConn1 -- 890/LConn1
  890/LConn3 -- Config13/RConn3
  Config13/LConn3 -- 888/RConn3
  Config13/LConn1 -- 888/RConn1
  Config13/LConn2 -- 888/RConn2
  Spot 890/RConn2 -- 890/RConn2
  Spot 890/RConn1 -- 890/RConn1
  Spot 890/RConn3 -- 890/RConn3
  DL_862-838/RConn1 -- 838/RConn2
  Spot 840/RConn1 -- 840/RConn1
  Spot 840/RConn2 -- 840/RConn2
  Spot 840/RConn3 -- 840/RConn3
  DL_858-864/RConn1 -- 864/RConn1
  DL_856/RConn1 -- 856/RConn2
  DL_822/RConn1 -- 822/RConn1
  DL_810/RConn1 -- 810/RConn2
  DL_826/RConn1 -- 826/RConn2
  Spot 848/RConn1 -- 848/RConn1 -- Shunt Capacitor3/LConn1
  Spot 848/RConn2 -- 848/RConn2 -- Shunt Capacitor4/LConn1
  Spot 848/RConn3 -- 848/RConn3 -- Shunt Capacitor5/LConn1
  Ground1/LConn1 -- 822/LConn2 -- 822/LConn3
  820/LConn2 -- Ground2/LConn1 -- 820/LConn3
  Ground6/LConn1 -- 818/LConn2 -- 818/LConn3
  Ground9/LConn1 -- 826/LConn1 -- 826/LConn3
  Ground10/LConn1 -- 810/RConn3 -- 810/RConn1
  Ground11/LConn1 -- 856/LConn3 -- 856/LConn1
  Ground12/LConn1 -- 864/LConn2 -- 864/LConn3
  Ground14/LConn1 -- 838/RConn1 -- 838/RConn3
  834/RConn2 -- DL_834 D-Z/RConn2 -- Config21/LConn2 -- Config18/RConn2
  834/RConn1 -- DL_834 D-Z/RConn1 -- Config21/LConn1 -- Config18/RConn1
  834/RConn3 -- Config18/RConn3 -- DL_834 D-Z/RConn3 -- Config21/LConn3
  RG10/RConn3 -- Config301/LConn3
  RG10/RConn2 -- Config301/LConn2
  RG10/RConn1 -- Config301/LConn1
  "852 "/LConn1 -- Config16/LConn1
  "852 "/LConn2 -- Config16/LConn2
  "852 "/LConn3 -- Config16/LConn3
  RG11/RConn1 -- Config5/RConn1
  RG11/RConn2 -- Config5/RConn2
  RG11/RConn3 -- Config5/RConn3
  Three-Phase Transformer (Two Windings)1/RConn2 -- XF10/LConn2
  XF10/LConn1 -- Three-Phase Transformer (Two Windings)1/RConn1
  XF10/LConn3 -- Three-Phase Transformer (Two Windings)1/RConn3
  XF10/RConn2 -- 888/LConn2
  XF10/RConn1 -- 888/LConn1
  XF10/RConn3 -- 888/LConn3
  Regulator 1/LConn2 -- 814/RConn2
  Regulator 1/LConn1 -- 814/RConn1
  Regulator 1/LConn3 -- 814/RConn3
  Regulator 1/RConn1 -- RG10/LConn1
  Regulator 1/RConn2 -- RG10/LConn2
  Regulator 1/RConn3 -- RG10/LConn3
  Regulator 2/LConn1 -- "852 "/RConn1
  Regulator 2/LConn2 -- "852 "/RConn2
  Regulator 2/LConn3 -- "852 "/RConn3
  Regulator 2/RConn3 -- RG11/LConn3
  Regulator 2/RConn2 -- RG11/LConn2
  Regulator 2/RConn1 -- RG11/LConn1

== system IEEE34_PQload/SM_IEEE34/Config1 ==
  Config302 : spsSeriesRLCBranchLib/Series RLC Branch  LConnTagsString=__new0  RConnTagsString=__new0  BranchType=RL  Resistance=2.7995 * length/1.6  Inductance=1.4855 / (2*fNom*pi) * length/1.6  SetiL0=off  InitialCurrent=0  Capacitance=1e-6  Setx0=off  InitialVoltage=0  Measurements=None
  Ground2 : spsGroundLib/Ground  LConnTagsString=a
  Ground3 : spsGroundLib/Ground  LConnTagsString=a
  Series RLC Branch2 : spsSeriesRLCBranchLib/Series RLC Branch  LConnTagsString=__new0  RConnTagsString=__new0  BranchType=C  Resistance=1  Inductance=1e-3  SetiL0=off  InitialCurrent=0  Capacitance=(4.2251*1e-6) / (2*fNom*pi) * length/1.6 / 2  Setx0=off  InitialVoltage=0  Measurements=None
  Series RLC Branch3 : spsSeriesRLCBranchLib/Series RLC Branch  LConnTagsString=__new0  RConnTagsString=__new0  BranchType=C  Resistance=1  Inductance=1e-3  SetiL0=off  InitialCurrent=0  Capacitance=(4.2251*1e-6) / (2*fNom*pi) * length/1.6 / 2  Setx0=off  InitialVoltage=0  Measurements=None
  a : PMIOPort  Tag=PMCPort  Side=Left
  "a " : PMIOPort  Tag=PMCPort  Port=2  Side=Right
  connections:
  Series RLC Branch3/RConn1 -- Ground3/LConn1
  Series RLC Branch2/RConn1 -- Ground2/LConn1
  Series RLC Branch2/LConn1 -- "a "/RConn1 -- Config302/RConn1
  Series RLC Branch3/LConn1 -- a/RConn1 -- Config302/LConn1
